simulink model "Multiagent_1030_ActorCritic"  (R2023a)
settings: Solver=FixedStepAuto  StartTime=0.0  StopTime=500  FixedStep=0.001  RelTol=1e-3
values from neighbouring files (symbols this model uses):
  INT_1 = [0;0.5;0]    [Paramaters.m]
  INT_2 = [-3.5;6;0]    [Paramaters.m]
  INT_3 = [-7.1;10;0.0]    [Paramaters.m]
  INT_4 = [-10.5;15;0.2]    [Paramaters.m]
  INT_5 = [-14;20;0.4]    [Paramaters.m]
(part 2 of 2)

== matlab function Multiagent_1030_ActorCritic/Subsystem7/Dynamics ==
  settings: updateMethod=DISCRETE
  data: t input; tau input; v input; v_dot output
    function v_dot = fcn(t,tau,v)
M = [25.8,0,0;0,33.8,1.0948;0,1.0948,2.76];
C = [0,0,-33.8*v(2)-1.0948*v(3);...
    0,0,25.8*v(1);...
    33.8*v(2)+1.0948*v(3),-25.8*v(1),0];
D = [0.7225 + 1.3274*abs(v(1)) + 5.8664*v(1)^2,0,0;...
     0,0.8612+36.2823*abs(v(1)) + 0.805*abs(v(3)),-0.1079 + 0.845*abs(v(1)) + 3.45*abs(v(3));...
     0,-0.1052 - 5.0437*abs(v(1)) - 0.13*abs(v(3)),1.9-0.08*abs(v(2))+0.75*abs(v(3))];

%M = [20,0,0;0,19,0.72;0,0.72,2.7];
% C = [0,0,-19*v(2)-0.72*v(3);0,0,20*v(1);19*v(2)+0.72*v(3),-20*v(1),0];
% 
% D = [0.72+1.3*abs(v(1))+5.8*v(1)^2,0,0;...
% 0,0.86+36*abs(v(2))+3*abs(v(3)),-0.1-2*abs(v(2))+2*abs(v(3));...
% 0,-0.1-5*abs(v(2))+3*abs(v(3)),6+4*abs(v(2))+4*abs(v(3))];

% tau_w=[3-0.2*sin(0.1*t)+0.1*cos(0.02*t)+0.1*rand(1);...
%     - 2.5 + 0.1*cos(0.1*t) + 0.1*sin(0.02*t) + 0.1*rand(1);...
%     3 - 0.2*sin(0.1*t) - 0.1*cos(0.02*t) + 0.1*rand(1)];

if (t < 15)
    flag = 1;
else 
    flag = 0;
end
noise = zeros(3,1);
% noise(1) = (50*sin(25*t) + 65*sin(45*(t-1)) + 45*sin(20*(t-0.5)) + 55*sin(35*(t-1.5)))*flag;
% noise(2) = (20*sin(25*t) + 10*sin(45*(t-1)) + 16*sin(20*(t-0.5)) + 20*sin(35*(t-1.5)))*flag;
% noise(3) = (9*sin(25*t) + 10*sin(45*(t-1)) + 14*sin(20*(t-0.5)) + 30*sin(35*(t-1.5)))*flag;

noise(1) = (10*sin(25*t) + 16*sin(45*(t-1)) + 15*sin(20*(t-0.5)) + 10*sin(35*(t-1.5)))*flag;
noise(2) = (50*sin(25*t) + 50*sin(45*(t-1)) + 40*sin(20*(t-0.5)) + 50*sin(35*(t-1.5)))*flag;
noise(3) = (40*sin(25*t) + 30*sin(45*(t-1)) + 45*sin(20*(t-0.5)) + 40*sin(35*(t-1.5)))*flag/20;

v_dot = -M\C*v-M\D*v+M\(tau  + noise);

== matlab function Multiagent_1030_ActorCritic/Subsystem7/Kinematics ==
  data: v input; eta_dot output; eta input
function eta_dot = fcn(v,eta)
J = [cos(eta(3)),-sin(eta(3)),0;sin(eta(3)),cos(eta(3)),0;0,0,1];
eta_dot = J*v;

== matlab function Multiagent_1030_ActorCritic/Subsystem7/Kinematics Controller/MATLAB Function1 ==
  data: e1 input; e2 input; e1_dot input; e2_dot input; gamma input; gamma_dot input; eta_r_dot input; e input; v_d output; eta input; z output
function [v_d,z] = fcn(e1,e2,e1_dot,e2_dot,gamma,gamma_dot,eta_r_dot,e,eta)
z=zeros(3,1);
b=zeros(3,1);
for k=1:3
    b(k)=(e2(k)+e(k))/(gamma(k)*(e1(k)-e(k)));
end
for k=1:3
    z(k)=1/2*log((e2(k)+e(k))/(gamma(k)*(e1(k)-e(k))));
end
p=0.5*(1./(e2+e)+1./(e1-e));
q=-0.5*(e2_dot./(e2_dot+e)-e1_dot./(e1_dot-e)-gamma_dot./gamma);
Phi_1=1/p(1)*(-z(1)+q(1)) + eta_r_dot(1);
Phi_2=1/p(2)*(-0.5*z(2)+q(2)) + eta_r_dot(2);
v_d = [Phi_1*cos(eta(3))+Phi_2*sin(eta(3));
      -Phi_1*sin(eta(3))+Phi_2*cos(eta(3));
      1/p(3)*(-z(3)+q(3))+eta_r_dot(3)];

== matlab function Multiagent_1030_ActorCritic/Subsystem7/Kinematics Controller/MATLAB Function4 ==
  data: eta_i_1_dot input; eta_r_dot output; eta_i_1 input; eta_r output
function [eta_r_dot,eta_r] = fcn(eta_i_1_dot,eta_i_1)
d=6;theta=2*pi/3;beta=0;
eta_d=[d*cos(theta);d*sin(theta);beta];
J=[cos(eta_i_1(3)),-sin(eta_i_1(3)),0;
    sin(eta_i_1(3)),cos(eta_i_1(3)),0;
    0,0,1];
J_dot=[-sin(eta_i_1(3))*eta_i_1_dot(3),-cos(eta_i_1(3))*eta_i_1_dot(3),0;
    cos(eta_i_1(3))*eta_i_1_dot(3),-sin(eta_i_1(3))*eta_i_1_dot(3),0;
    0,0,0];
eta_r=eta_i_1 + J*eta_d;
eta_r_dot=eta_i_1_dot + J_dot*eta_d;

== matlab function Multiagent_1030_ActorCritic/Subsystem7/RL controller/MATLAB Function ==
  settings: updateMethod=DISCRETE
  data: v input; v_dot input; eta_r input; eta_r_dot input; v_d input; tau output; v_d_dot input; z input; Wc input; Wa input; u input; tau_d output; u output; Wa_dot output; Wc_dot output
function [tau,tau_d,u,Wa_dot,Wc_dot] = fcn(v,v_dot,eta_r,eta_r_dot,v_d,v_d_dot,z,Wc,Wa,u)
%Q=eye(3);R=eye(3);
M = [25.8,0,0;0,33.8,1.0948;0,1.0948,2.76];
%M = [20,0,0;0,19,0.72;0,0.72,2.7];
invM = inv(M);
eta_c = 10;
eta_a1 = 10;
eta_a2 = 20;
nuy = 0.01;
GAMMA = 20; %%khong cap nhat
z2=v-v_d;
z2_dot=v_dot-v_d_dot;
x=[z2;z;eta_r;eta_r_dot];

gradPhi = [2*x(1),0,0;...
             x(2),x(1),0;...
             x(3),0,x(1);...
             0,2*x(2),0;...
             0,x(3),x(2);...
             0,0,2*x(3);...
              2*x(1)*x(7)^2,0,0;...
              0,2*x(2)*x(8)^2,0;...
              0,0,2*x(3)*x(9)^2;...
              2*x(1)*x(4)^2,0,0;...
              0,2*x(2)*x(5)^2,0;...
              0,0,2*x(3)*x(6)^2;...
              2*x(1)*x(10)^2,0,0;...
              0,2*x(2)*x(11)^2,0;...
              0,0,2*x(3)^2*x(12)^2]; 
             %15x3
%Phi = [x(1)^2; x(1)*x(2); x(1)*x(3); x(2)^2; x(2)*x(3); x(3)^2; x(1)^2*x(7)^2; x(2)^2*x(8)^2; ...
%    x(3)^2*x(9)^2; x(1)^2*x(4)^2; x(2)^2*x(5)^2; x(3)^2*x(6)^2;x(1)^2*x(10)^2;x(2)^2*x(11)^2;x(3)^2*x(12)^2];
%J = [cos(eta(3)),-sin(eta(3)),0;sin(eta(3)),cos(eta(3)),0;0,0,1];
% J_dot = [-sin(eta(3))*v(3), -cos(eta(3))*v(3), 0;
%       cos(eta(3))*v(3), -sin(eta(3))*v(3), 0;
%              0, 0, 0];
% C_d = [0,0,-33.8*v(2)-1.0948*v(3);0,0,25.8*v(1);33.8*v(2)+1.0948*v(3),-25.8*v(1),0];
% D_d = [0.7225 + 1.3274*abs(v(1)) + 5.8664*v(1)^2,0,0;...
%      0,0.8612+36.2823*abs(v(1)) + 0.805*abs(v(3)),-0.1079 + 0.845*abs(v(1)) + 3.45*abs(v(3));...
%      0,-0.1052 - 5.0437*abs(v(1)) - 0.13*abs(v(3)),1.9-0.08*abs(v(2))+0.75*abs(v(3))];
C_d = [0,0,-33.8*v_d(2)-1.0948*v_d(3);0,0,25.8*v_d(1);33.8*v_d(2)+1.0948*v_d(3),-25.8*v_d(1),0];
D_d = [0.7225 + 1.3274*abs(v_d(1)) + 5.8664*v_d(1)^2,0,0;...
     0,0.8612+36.2823*abs(v_d(1)) + 0.805*abs(v_d(3)),-0.1079 + 0.845*abs(v_d(1)) + 3.45*abs(v_d(3));...
     0,-0.1052 - 5.0437*abs(v_d(1)) - 0.13*abs(v_d(3)),1.9-0.08*abs(v_d(2))+0.75*abs(v_d(3))];

% C_d = [0,0,-19*v_d(2)-0.72*v_d(3);0,0,20*v_d(1);19*v_d(2)+0.72*v_d(3),-20*v_d(1),0];
% D_d = [0.72+1.3*abs(v_d(1))+5.8*v_d(1)^2,0,0;...
% 0,0.86+36*abs(v_d(2))+3*abs(v_d(3)),-0.1-2*abs(v_d(2))+2*abs(v_d(3));...
% 0,-0.1-5*abs(v_d(2))+3*abs(v_d(3)),6+4*abs(v_d(2))+4*abs(v_d(3))];


zigma=gradPhi*z2_dot;
delta_hjb=Wc'*zigma + z2'*z2 + u'*u;
Wc_dot = -eta_c*GAMMA*zigma/(1+nuy*(zigma'*GAMMA*zigma))*delta_hjb;
Wa_dot = -eta_a1/sqrt(1+zigma'*zigma)*gradPhi*(invM*invM')*gradPhi'*(Wa-Wc)*delta_hjb-eta_a2*(Wa-Wc);

tau_d = M*v_d_dot+C_d*v_d+D_d*v_d;

u = -1/2*invM'*gradPhi'*Wa;

tau = tau_d + u;

== matlab function Multiagent_1030_ActorCritic/eta_0/MATLAB Function ==
  data: t input; eta_r output; eta_r_dot output
function [eta_r,eta_r_dot] = fcn(t)

if t<40
    eta_n_1 = [0.5*t;0;0];
else
    eta_n_1 = [0.5*40 + 50*sin(0.01*(t-40));50*(1-cos(0.01*(t-40)));0.01*(t-40)];
end
eta_r = eta_n_1;
if t<40
    eta_n_1_dot = [0.5;0;0];
else
    eta_n_1_dot = [0.5*cos(0.01*(t-40));0.5*sin(0.01*(t-40));0.01];
end
eta_r_dot=eta_n_1_dot;


%     eta_n_1 = [60*sin(0.05*t) + 40*cos(0.05*t) - 35; -60*sin(0.05*t) + 40*sin(0.05*t) + t + 75;0.05*t];
% eta_r = eta_n_1;
%     eta_n_1_dot = [3*cos(0.05*t) - 2*sin(0.05*t);-3*sin(0.05*t) + 2*cos(0.05*t) + 1;0.05];
% eta_r_dot=eta_n_1_dot;

== matlab function Multiagent_1030_ActorCritic/Subsystem2/MATLAB Function2 ==
  data: t input; e1 output; e2 output; e1_dot output; e2_dot output; gamma output; gamma_dot output
function [e1,e2,e1_dot,e2_dot,gamma,gamma_dot] = fcn(t)
% e1=[1.4*exp(-0.05*t)+0.1;0.9*exp(-0.04*t)+0.1;exp(-0.1*t)+0.05];
% e2=[0.9*exp(-0.05*t)+0.1;1.4*exp(-0.04*t)+0.1;exp(-0.1*t)+0.05];
% e1_dot=[1.4*(-0.05)*exp(-0.05*t);0.9*(-0.04)*exp(-0.04*t);-0.035*exp(-0.1*t)];
% e2_dot=[-0.9*0.05*exp(-0.05*t);-1.4*0.04*exp(-0.04*t);-0.035*exp(-0.1*t)];

e1=[1.4*exp(-0.05*t)+0.1;0.9*exp(-0.04*t)+0.1;exp(-0.1*t)+0.05];
e2=[0.9*exp(-0.05*t)+0.1;1.4*exp(-0.04*t)+0.1;exp(-0.1*t)+0.05];
e1_dot=[2.4*(-0.05)*exp(-0.05*t);0.9*(-0.04)*exp(-0.04*t);-0.035*exp(-0.1*t)];
e2_dot=[-1.9*0.05*exp(-0.05*t);-1.4*0.04*exp(-0.04*t);-0.035*exp(-0.1*t)];
gamma=e2./e1;
gamma_dot=(e2_dot.*e1_dot - e1_dot.*e2_dot)./(e2_dot.^2);

== matlab function Multiagent_1030_ActorCritic/MATLAB Function ==
  data: input input; v output; w output
function [v,w] = fcn(input)

v = sqrt(input(1)^2+input(2)^2);
w = input(3);
end

== matlab function Multiagent_1030_ActorCritic/Subsystem1/Kinematics Controller/MATLAB Function1 ==
  data: e1 input; e2 input; e1_dot input; e2_dot input; gamma input; gamma_dot input; eta_r_dot input; e input; v_d output; eta input; z output
function [v_d,z] = fcn(e1,e2,e1_dot,e2_dot,gamma,gamma_dot,eta_r_dot,e,eta)
z=zeros(3,1);
b=zeros(3,1);
for k=1:3
    b(k)=(e2(k)+e(k))/(gamma(k)*(e1(k)-e(k)));
end
for k=1:3
    z(k)=1/2*log((e2(k)+e(k))/(gamma(k)*(e1(k)-e(k))));
end
p=0.5*(1./(e2+e)+1./(e1-e));
q=-0.5*(e2_dot./(e2_dot+e)-e1_dot./(e1_dot-e)-gamma_dot./gamma);
Phi_1=1/p(1)*(-z(1)+q(1)) + eta_r_dot(1);
Phi_2=1/p(2)*(-0.5*z(2)+q(2)) + eta_r_dot(2);
v_d = [Phi_1*cos(eta(3))+Phi_2*sin(eta(3));
      -Phi_1*sin(eta(3))+Phi_2*cos(eta(3));
      1/p(3)*(-z(3)+q(3))+eta_r_dot(3)];

== matlab function Multiagent_1030_ActorCritic/Subsystem/Kinematics ==
  data: v input; eta_dot output; eta input
function eta_dot = fcn(v,eta)
J = [cos(eta(3)),-sin(eta(3)),0;sin(eta(3)),cos(eta(3)),0;0,0,1];
eta_dot = J*v;

== matlab function Multiagent_1030_ActorCritic/Subsystem/RL controller/Controller ==
  data: tau output; tau_d output; u output; v input; v_dot input; eta_r input; Wa_dot output; Wc_dot output; eta_r_dot input; v_d input; v_d_dot input; z input; Wc input; Wa input; u input; R output; RL parameter
function [tau,tau_d,u,Wa_dot,Wc_dot,R] = fcn(v,v_dot,eta_r,eta_r_dot,v_d,v_d_dot,z,Wc,Wa,u,RL)

%Q=eye(3);R=eye(3);
M = [25.8,0,0;0,33.8,1.0948;0,1.0948,2.76];
%M = [20,0,0;0,19,0.72;0,0.72,2.7];
invM = inv(M);
eta_c = 10;
eta_a1 = 10;
eta_a2 = 20;
nuy = 0.01;
GAMMA = 20; %%khong cap nhat
z2=v-v_d;
z2_dot=v_dot-v_d_dot;
x=[z2;z;eta_r;eta_r_dot];

gradPhi = [2*x(1),0,0;...
             x(2),x(1),0;...
             x(3),0,x(1);...
             0,2*x(2),0;...
             0,x(3),x(2);...
             0,0,2*x(3);...
              2*x(1)*x(7)^2,0,0;...
              0,2*x(2)*x(8)^2,0;...
              0,0,2*x(3)*x(9)^2;...
              2*x(1)*x(4)^2,0,0;...
              0,2*x(2)*x(5)^2,0;...
              0,0,2*x(3)*x(6)^2;...
              2*x(1)*x(10)^2,0,0;...
              0,2*x(2)*x(11)^2,0;...
              0,0,2*x(3)^2*x(12)^2]; 
             %15x3
% Phi = [x(1)^2; x(1)*x(2); x(1)*x(3); x(2)^2; x(2)*x(3); x(3)^2; x(1)^2*x(7)^2; x(2)^2*x(8)^2; ...
%     x(3)^2*x(9)^2; x(1)^2*x(4)^2; x(2)^2*x(5)^2; x(3)^2*x(6)^2;x(1)^2*x(10)^2;x(2)^2*x(11)^2;x(3)^2*x(12)^2];
%J = [cos(eta(3)),-sin(eta(3)),0;sin(eta(3)),cos(eta(3)),0;0,0,1];
% J_dot = [-sin(eta(3))*v(3), -cos(eta(3))*v(3), 0;
%       cos(eta(3))*v(3), -sin(eta(3))*v(3), 0;
%              0, 0, 0];
% C_d = [0,0,-33.8*v(2)-1.0948*v(3);0,0,25.8*v(1);33.8*v(2)+1.0948*v(3),-25.8*v(1),0];
% D_d = [0.7225 + 1.3274*abs(v(1)) + 5.8664*v(1)^2,0,0;...
%      0,0.8612+36.2823*abs(v(1)) + 0.805*abs(v(3)),-0.1079 + 0.845*abs(v(1)) + 3.45*abs(v(3));...
%      0,-0.1052 - 5.0437*abs(v(1)) - 0.13*abs(v(3)),1.9-0.08*abs(v(2))+0.75*abs(v(3))];
C_d = [0,0,-33.8*v_d(2)-1.0948*v_d(3);0,0,25.8*v_d(1);33.8*v_d(2)+1.0948*v_d(3),-25.8*v_d(1),0];
D_d = [0.7225 + 1.3274*abs(v_d(1)) + 5.8664*v_d(1)^2,0,0;...
     0,0.8612+36.2823*abs(v_d(1)) + 0.805*abs(v_d(3)),-0.1079 + 0.845*abs(v_d(1)) + 3.45*abs(v_d(3));...
     0,-0.1052 - 5.0437*abs(v_d(1)) - 0.13*abs(v_d(3)),1.9-0.08*abs(v_d(2))+0.75*abs(v_d(3))];

% C_d = [0,0,-19*v_d(2)-0.72*v_d(3);0,0,20*v_d(1);19*v_d(2)+0.72*v_d(3),-20*v_d(1),0];
% D_d = [0.72+1.3*abs(v_d(1))+5.8*v_d(1)^2,0,0;...
% 0,0.86+36*abs(v_d(2))+3*abs(v_d(3)),-0.1-2*abs(v_d(2))+2*abs(v_d(3));...
% 0,-0.1-5*abs(v_d(2))+3*abs(v_d(3)),6+4*abs(v_d(2))+4*abs(v_d(3))];

% V = Wc'*Phi; 
zigma=gradPhi*z2_dot;
delta_hjb=Wc'*zigma + z2'*z2 + u'*u;
Wc_dot = -eta_c*GAMMA*zigma/(1+nuy*(zigma'*GAMMA*zigma))*delta_hjb;
Wa_dot = -eta_a1/sqrt(1+zigma'*zigma)*gradPhi*(invM*invM')*gradPhi'*(Wa-Wc)*delta_hjb-eta_a2*(Wa-Wc);

tau_d = M*v_d_dot+C_d*v_d+D_d*v_d;

u = -1/2*invM'*gradPhi'*Wa;

if (RL == 0)
    u = [0;0;0];
end

tau = tau_d + u;

Q = [eye(6) zeros(6,6); zeros(6,6) zeros(6)];
R = x'*Q*x + (tau_d + u)'*(tau_d + u);
